simulink model "Copy_of_simpleDemonstrationDouble"  (R2023a)
settings: Solver=VariableStepAuto  StartTime=0.0  StopTime=Tstep*ofdmSymLen*6  RelTol=1e-3
PreLoadFcn:
  | % 100 MHz scenario
  | scs = 30e3;
  | fftLength = 4096;
  | NSubcarriers = 3276;
  | cpLength = 288;
  | windowLength = 20;
  | 
  | nGuardBandCarrier = fftLength - NSubcarriers;
  | ofdmSymLen = fftLength+cpLength;
  | overSamplingRate = 7;
  | filterLength = 6*70;
  | 
  | BW = scs*fftLength;                       %  Signal BW
  | Tstep = 1/BW;                   %  Simulation BW BB
  | RF = 3.7e9;                       %  RF center frequency
  | IF = 500e6;                          % IF frequency
  | dataRatePA = 1/BW;  % PA characterization sample time
  | N = nGuardBandCarrier/2;
  | HPF_cutoff = RF - 500e6;
  | 
  | bw = 100e6;
  | [txWaveform, sampleRate] = helperPACharGenerateOFDM(bw);
  | 
  | dataFileName = sprintf("helperPACharSavedData%dMHz",bw/1e6);
  | load(dataFileName,"results")
  | paInput = results.InputWaveform;
  | paOutput = results.OutputWaveform;
  | modType = 'memPoly';
  | memLen = 5;
  | degLen = 5;
  | halfDataPts = round(length(paInput)/2);
  | origState = warning;
  | warning('off', 'MATLAB:rankDeficientMatrix')
  | paModelMemPoly = double(helperPACharMemPolyModel('coefficientFinder', ...
  |   paInput(1:halfDataPts),paOutput(1:halfDataPts),memLen,degLen,modType));
  | warning(origState);
  | 
  | gain = results.LinearGain;
  | scaleFactor = double(max(abs(paOutput))/max(abs(txWaveform))/gain);
InitFcn:
  | % Initialize model parameters
  | NRInfo = get_param([gcs '/5G NR Test Model'], 'UserData');
  | MultirateBlock = [gcs '/Multirate Parameters'];
  | hInitializeNRTMModel(MultirateBlock,NRInfo);
StopFcn:
  | clear hDecodeSubframe;
undefined symbols (not defined in the file or in its folder): errorPDec, errorPInt, errorStDec, errorStInt, firceqrip, modNFloor, nDec, nInt, OSR, Probability, S, waveform
libraries: simrfV2elements x20, simrfV2util1 x11, simrfV2_lib x5, dspstat3 x4, simrfV2systems x3, commofdm x2, commrfcorlib x2, dspmlti4 x2, simrfV2junction1 x2, commrandsrc3 x1, commdigbbndam3 x1, commutil2 x1
(part 1 of 2)
settings Model: SimulationMode=accelerator  Creator=Hossein  LastModifiedBy=Hossein

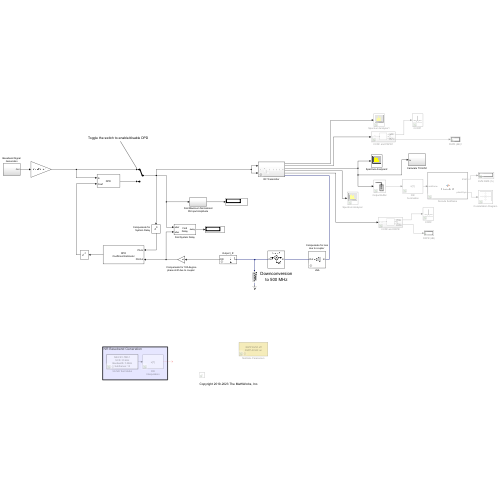
[thumbnail: Simulink's stored preview of the top-level diagram]
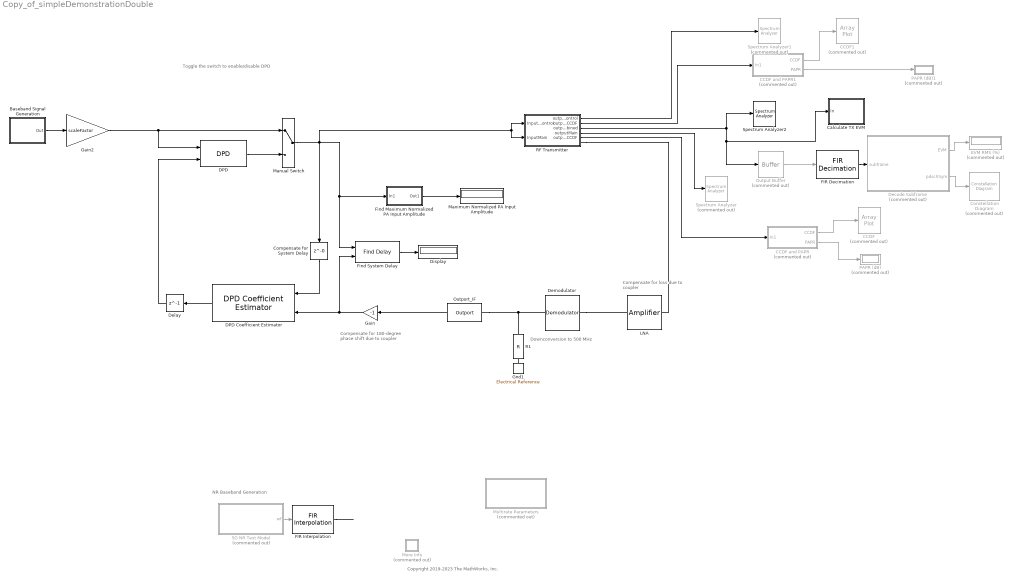
== system Copy_of_simpleDemonstrationDouble ==
  note: Copyright 2019-2023 The MathWorks, Inc.
  note: Downconversion
      | to 500 MHz
  note: Toggle the switch to enable/disable DPD
  note: Compensate for 180-degree
      | phase shift due to coupler
  note: Compensate for loss
      | due to coupler
  note: NR Baseband Generation
  5G NR Test Model : MATLAB Function  Tag=BlockGeneratedWWGApp  Commented=on  TreatAsAtomicUnit=on  SystemSampleTime=1.3020833333333333957e-07  mask(5G NR Test Model Waveform Generator){nsamps=1, OutputAfterFinalValue=Cyclic repetition}
      mask prompts: nsamps "Samples per frame:"; OutputAfterFinalValue "Form output after final data value by:"
      mask init:
      | %% Generating NR Test Models waveform
      | % NR Test Models configuration
      | cfgDLTM = nrDLCarrierConfig;
      | cfgDLTM.Label = 'NR-FR1-TM3.1';
      | cfgDLTM.FrequencyRange = 'FR1';
      | cfgDLTM.ChannelBandwidth = 5;
      | cfgDLTM.NCellID = 1;
      | cfgDLTM.NumSubframes = 10;
      | cfgDLTM.WindowingPercent = 0;
      | cfgDLTM.SampleRate = [];
      | cfgDLTM.CarrierFrequency = 0;
      | 
      | %% SCS specific carriers
      | scscarrier = nrSCSCarrierConfig;
      | scscarrier.SubcarrierSpacing = 30;
      | scscarrier.NSizeGrid = 11;
      | scscarrier.NStartGrid = 0;
      | 
      | cfgDLTM.SCSCarriers = {scscarrier};
      | 
      | %% Bandwidth Parts
      | bwp = nrWavegenBWPConfig;
      | bwp.BandwidthPartID = 1;
      | bwp.Label = 'BWP1';
      | bwp.SubcarrierSpacing = 30;
      | bwp.CyclicPrefix = 'normal';
      | bwp.NSizeBWP = 11;
      | bwp.NStartBWP = 0;
      | 
      | cfgDLTM.BandwidthParts = {bwp};
      | 
      | %% Synchronization Signals Burst
      | ssburst = nrWavegenSSBurstConfig;
      | ssburst.Enable = false;
      | ssburst.Power = 0;
      | ssburst.BlockPattern = 'Case A';
      | ssburst.TransmittedBlocks = [1 0 0 0];
      | ssburst.Period = 10;
      | ssburst.NCRBSSB = [];
      | ssburst.KSSB = 0;
      | ssburst.DataSource = 'MIB';
      | ssburst.DMRSTypeAPosition = 2;
      | ssburst.CellBarred = false;
      | ssburst.IntraFreqReselection = false;
      | ssburst.PDCCHConfigSIB1 = 0;
      | ssburst.SubcarrierSpacingCommon = 30;
      | 
      | cfgDLTM.SSBurst = ssburst;
      | 
      | %% CORESET and Search Space Configuration
      | coreset = nrCORESETConfig;
      | coreset.CORESETID = 1;
      | coreset.Label = 'CORESET1';
      | coreset.FrequencyResources = 1;
      | coreset.Duration = 2;
      | coreset.CCEREGMapping = 'noninterleaved';
      | coreset.REGBundleSize = 2;
      | coreset.InterleaverSize = 2;
      | coreset.ShiftIndex = 0;
      | coreset.PrecoderGranularity = 'sameAsREG-bundle';
      | coreset.RBOffset = [];
      | 
      | cfgDLTM.CORESET = {coreset};
      | 
      | % Search Spaces
      | searchspace = nrSearchSpaceConfig;
      | searchspace.SearchSpaceID = 1;
      | searchspace.Label = 'SearchSpace1';
      | searchspace.CORESETID = 1;
      | searchspace.SearchSpaceType = 'common';
      | searchspace.StartSymbolWithinSlot = 0;
      | searchspace.SlotPeriodAndOffset = [1 0];
      | searchspace.Duration = 1;
      | searchspace.NumCandidates = [8 8 0 0 0];
      | 
      | cfgDLTM.SearchSpaces = {searchspace};
      | 
      | %% PDCCH Instances Configuration
      | pdcch = nrWavegenPDCCHConfig;
      | pdcch.Enable = true;
      | pdcch.Label = 'PDCCH1';
      | pdcch.Power = 0;
      | pdcch.BandwidthPartID = 1;
      | pdcch.SearchSpaceID = 1;
      | pdcch.AggregationLevel = 1;
      | pdcch.AllocatedCandidate = 1;
      | pdcch.CCEOffset = [];
      | pdcch.SlotAllocation = 0;
      | pdcch.Period = 1;
      | pdcch.Coding = false;
      | pdcch.DataBlockSize = 20;
      | pdcch.DataSource = 'PN23';
      | pdcch.RNTI = 0;
      | pdcch.DMRSScramblingID = 1;
      | pdcch.DMRSPower = 0;
      | 
      | cfgDLTM.PDCCH = {pdcch};
      | 
      | %% PDSCH Instances Configuration
      | % PDSCH 1
      | pdsch1 = nrWavegenPDSCHConfig;
      | pdsch1.Enable = true;
      | pdsch1.Label = 'Partial band PDSCH sequence with 64QAM modulation scheme (target, RNTI = 0)';
      | pdsch1.Power = 0;
      | pdsch1.BandwidthPartID = 1;
      | pdsch1.Modulation = '64QAM';
      | pdsch1.NumLayers = 1;
      | pdsch1.MappingType = 'A';
      | pdsch1.ReservedCORESET = [];
      | pdsch1.SymbolAllocation = [0 14];
      | pdsch1.SlotAllocation = 0;
      | pdsch1.Period = 1;
      | pdsch1.PRBSet = 3:10;
      | pdsch1.VRBToPRBInterleaving = 0;
      | pdsch1.VRBBundleSize = 2;
      | pdsch1.NID = [];
      | pdsch1.RNTI = 0;
      | pdsch1.Coding = false;
      | pdsch1.TargetCodeRate = 0.4785;
      | pdsch1.TBScaling = 1;
      | pdsch1.XOverhead = 0;
      | pdsch1.RVSequence = 0;
      | pdsch1.DataSource = 'PN23';
      | pdsch1.DMRSPower = 0;
      | pdsch1.EnablePTRS = false;
      | pdsch1.PTRSPower = 0;
      | 
      | % PDSCH Reserved PRB
      | pdsch1ReservedPRB = nrPDSCHReservedConfig;
      | pdsch1ReservedPRB.PRBSet = 0:2;
      | pdsch1ReservedPRB.SymbolSet = [0 1];
      | pdsch1ReservedPRB.Period = 1;
      | 
      | pdsch1.ReservedPRB = {pdsch1ReservedPRB};
      | 
      | % PDSCH DM-RS
      | pdsch1DMRS = nrPDSCHDMRSConfig;
      | pdsch1DMRS.DMRSConfigurationType = 1;
      | pdsch1DMRS.DMRSReferencePoint = 'CRB0';
      | pdsch1DMRS.DMRSTypeAPosition = 2;
      | pdsch1DMRS.DMRSAdditionalPosition = 1;
      | pdsch1DMRS.DMRSLength = 1;
      | pdsch1DMRS.CustomSymbolSet = [];
      | pdsch1DMRS.DMRSPortSet = [];
      | pdsch1DMRS.NIDNSCID = [];
      | pdsch1DMRS.NSCID = 0;
      | pdsch1DMRS.NumCDMGroupsWithoutData = 1;
      | pdsch1DMRS.DMRSDownlinkR16 = 0;
      | 
      | pdsch1.DMRS = pdsch1DMRS;
      | 
      | % PDSCH PT-RS
      | pdsch1PTRS = nrPDSCHPTRSConfig;
      | pdsch1PTRS.TimeDensity = 4;
      | pdsch1PTRS.FrequencyDensity = 2;
      | pdsch1PTRS.REOffset = '00';
      | pdsch1PTRS.PTRSPortSet = [];
      | 
      | pdsch1.PTRS = pdsch1PTRS;
      | 
      | % PDSCH 2
      | pdsch2 = nrWavegenPDSCHConfig;
      | pdsch2.Enable = true;
      | pdsch2.Label = 'Partial band PDSCH sequence with 64QAM modulation scheme (target, RNTI = 2)';
      | pdsch2.Power = 0;
      | pdsch2.BandwidthPartID = 1;
      | pdsch2.Modulation = '64QAM';
      | pdsch2.NumLayers = 1;
      | pdsch2.MappingType = 'A';
      | pdsch2.ReservedCORESET = [];
      | pdsch2.SymbolAllocation = [2 12];
      | pdsch2.SlotAllocation = 0;
      | pdsch2.Period = 1;
      | pdsch2.PRBSet = 0:2;
      | pdsch2.VRBToPRBInterleaving = 0;
      | pdsch2.VRBBundleSize = 2;
      | pdsch2.NID = [];
      | pdsch2.RNTI = 2;
      | pdsch2.Coding = false;
      | pdsch2.TargetCodeRate = 0.4785;
      | pdsch2.TBScaling = 1;
      | pdsch2.XOverhead = 0;
      | pdsch2.RVSequence = 0;
      | pdsch2.DataSource = 'PN23';
      | pdsch2.DMRSPower = 0;
      | pdsch2.EnablePTRS = false;
      | pdsch2.PTRSPower = 0;
      | 
      | pdschreserved = nrPDSCHReservedConfig;
      | pdschreserved.PRBSet = 0:2;
      | pdschreserved.SymbolSet = [0 1];
      | pdschreserved.Period = 1;
      | 
      | pdsch2.ReservedPRB = {pdschreserved};
      | 
      | pdschdmrs = nrPDSCHDMRSConfig;
      | pdschdmrs.DMRSConfigurationType = 1;
      | pdschdmrs.DMRSReferencePoint = 'CRB0';
      | pdschdmrs.DMRSTypeAPosition = 2;
      | pdschdmrs.DMRSAdditionalPosition = 1;
      | pdschdmrs.DMRSLength = 1;
      | pdschdmrs.CustomSymbolSet = [];
      | pdschdmrs.DMRSPortSet = [];
      | pdschdmrs.NIDNSCID = [];
      | pdschdmrs.NSCID = 0;
      | pdschdmrs.NumCDMGroupsWithoutData = 1;
      | pdschdmrs.DMRSDownlinkR16 = 0;
      | 
      | pdsch2.DMRS = pdschdmrs;
      | 
      | pdschptrs = nrPDSCHPTRSConfig;
      | pdschptrs.TimeDensity = 4;
      | pdschptrs.FrequencyDensity = 2;
      | pdschptrs.REOffset = '00';
      | pdschptrs.PTRSPortSet = [];
      | 
      | pdsch2.PTRS = pdschptrs;
      | 
      | cfgDLTM.PDSCH = {pdsch1,pdsch2};
      | 
      | %% CSI-RS Instances Configuration
      | csirs = nrWavegenCSIRSConfig;
      | csirs.Enable = false;
      | csirs.Label = 'CSIRS1';
      | csirs.Power = 0;
      | csirs.BandwidthPartID = 1;
      | csirs.CSIRSType = 'nzp';
      | csirs.CSIRSPeriod = 'on';
      | csirs.RowNumber = 1;
      | csirs.Density = 'three';
      | csirs.SymbolLocations = 0;
      | csirs.SubcarrierLocations = 0;
      | csirs.NumRB = 11;
      | csirs.RBOffset = 0;
      | csirs.NID = 1;
      | 
      | cfgDLTM.CSIRS = {csirs};
      | 
      | % Generation
      | [waveform,info] = nrWaveformGenerator(cfgDLTM);
      | 
      | Fs = info.ResourceGrids(1).Info.SampleRate; 								 % Specify the sample rate of the waveform in Hz
      | 
      | %% Configuring block: update parameters and UserData
      | % Get current block
      | thisBlock = gcb;
      | 
      | % Set info parameters
      | maskHandle = Simulink.Mask.get(thisBlock);
      | textFsDialog = maskHandle.getDialogControl('textFs');
      | textFsDialog.Prompt = ['Waveform sample rate (Fs): ' num2str(Fs*1e-6,'%.9g') ' MHz'];
      | textWfLengthDialog = maskHandle.getDialogControl('textWFLength');
      | textWfLengthDialog.Prompt = ['Waveform length: ' num2str(length(waveform)) ' samples'];
      | 
      | % Set sample time of the block
      | set_param(thisBlock, 'SystemSampleTime', num2str(nsamps/Fs,'%.20g'));
      | 
      | % Update UserData
      | outVar.WaveformConfig = cfgDLTM;
      | outVar.WaveformLength = length(waveform);
      | outVar.Fs = Fs;
      | set_param(thisBlock, 'UserData', outVar);
  Baseband Signal Generation : Subsystem
  CCDF : ArrayPlot  Commented=on  WindowPosition=[823.000000,372.000000,866.000000,486.000000,]  ScopeFrameLocation=window  SampleIncrement=0.1  XOffset=-40.7414  YScale=Log  PlotType=Line  Title=CCDF Curve  XLabel=Rel Power (dB)  YLabel=Probability (%)  YLimits=[-12.4981,112.4829]  ShowLegend=on
  CCDF and PAPR : Subsystem  Commented=on
  CCDF and PAPR1 : Subsystem  Commented=on
  CCDF1 : ArrayPlot  Commented=on  WindowPosition=[823.000000,372.000000,866.000000,486.000000,]  ScopeFrameLocation=window  SampleIncrement=0.1  XOffset=-40.7414  YScale=Log  PlotType=Line  Title=CCDF Curve  XLabel=Rel Power (dB)  YLabel=Probability (%)  YLimits=[-12.498,112.4823]  ShowLegend=on
  Calculate TX EVM : Subsystem
  Compensate for System Delay : Delay  DelayLength=0
  Constellation Diagram : ConstellationDiagram  Commented=on  WindowPosition=[576.000000,404.000000,590.000000,412.000000,]  ScopeFrameLocation=window  ShowReferenceConstellation=off  DefaultConfigurationName=comm.scopes.ConstellationDiagramBlockCfg
  DPD : commrfcorlib/DPD  PolynomialType=Memory polynomial  CoefficientSource=Input port  Coefficients=complex([1 0 0 0 0; 0 0 0 0 0; 0 0 0 0 0])  SimulateUsing=Code generation
  DPD Coefficient Estimator : commrfcorlib/DPD Coefficient Estimator  DesiredAmplitudeGaindB=10*log10(gain)  PolynomialType=Memory polynomial  Degree=3  MemoryDepth=5  Algorithm=Recursive least squares  ForgettingFactorSource=Property  ForgettingFactor=0.999  InitialCoefficientEstimate=[]  SimulateUsing=Code generation
  Decode Subframe : MATLAB Function  Commented=on  TreatAsAtomicUnit=on
  Delay : Delay  DelayLength=1
  Demodulator : simrfV2systems/Demodulator  classname=rfdemod  Source_linear_gain=Available power gain  linear_gain=0 dB  Poly_Coeffs=[0 1]  LOFreq=RF-IF Hz  Zin=50  Zout=50  AddIRFilter=on  AddCSFilter=off  InternalGrounding=on  ForceNextInit=off  Source_Poly=Even and odd order  IPType=Input  IP2=inf dBm  IP3=inf dBm  P1dB=inf dBm  Psat=inf dBm  Gcomp=inf dBm  NF=1  Isolation=inf dB  AddPhaseNoise=off  PhaseNoiseOffset=[5e5 1e6 5e6]  PhaseNoiseLevel=[-108 -130 -140]  AutoImpulseLengthPN=on  ImpulseLengthPN=1e-10  ImpulseLength_unitPN=s  DesignMethodIR=Ideal  ResponseTypeIR=Highpass  ImplementationIR=LC Tee  ImplementationIdealIR=Constant per carrier  ImplementationRationalIR=Transfer function  UseFilterOrderIR=on  FilterOrderIR=3  PassFreq_lpIR=1  PassFreq_lp_unitIR=GHz  PassFreq_hpIR=HPF_cutoff  PassFreq_hp_unitIR=Hz  PassFreq_bpIR=[2 3]  PassFreq_bp_unitIR=GHz  PassFreq_bsIR=[1 4]  PassFreq_bs_unitIR=GHz  PassAttenIR=10*log10(2)  StopFreq_lpIR=2  StopFreq_lp_unitIR=GHz  StopFreq_hpIR=1  StopFreq_hp_unitIR=GHz  StopFreq_bpIR=[1.5 3.5]  StopFreq_bp_unitIR=GHz  StopFreq_bsIR=[2.1 2.9]  StopFreq_bs_unitIR=GHz  StopAttenIR=40  RsrcIR=50  RloadIR=50  AutoImpulseLengthIR=on  ImpulseLengthIR=1e-10  ImpulseLength_unitIR=s  DesignMethodCS=Ideal  ResponseTypeCS=Lowpass  ImplementationCS=LC Tee  ImplementationIdealCS=Constant per carrier  ImplementationRationalCS=Transfer function  UseFilterOrderCS=on  FilterOrderCS=3  PassFreq_lpCS=1  PassFreq_lp_unitCS=GHz  PassFreq_hpCS=2  PassFreq_hp_unitCS=GHz  PassFreq_bpCS=[2 3]  PassFreq_bp_unitCS=GHz  PassFreq_bsCS=[1 4]  PassFreq_bs_unitCS=GHz  PassAttenCS=10*log10(2)  StopFreq_lpCS=2  StopFreq_lp_unitCS=GHz  StopFreq_hpCS=1  StopFreq_hp_unitCS=GHz  StopFreq_bpCS=[1.5 3.5]  StopFreq_bp_unitCS=GHz  StopFreq_bsCS=[2.1 2.9]  StopFreq_bs_unitCS=GHz  StopAttenCS=40  RsrcCS=50  RloadCS=50  AutoImpulseLengthCS=on  ImpulseLengthCS=1e-10  ImpulseLength_unitCS=s
  Display : Display
  EVM RMS (%) : Display  Commented=on
  FIR Decimation : dspmlti4/FIR Decimation  FilterSource=Dialog parameters  h=firceqrip(nDec,(NRInfo.Fs*1e-6/4)/(NRInfo.Fs*1e-6*OSR/2),[errorPDec errorStDec],'passedge')  D=OSR  filtStruct=Direct form  FilterObject=FDECIM  InputProcessing=Columns as channels (frame based)  framing=Enforce single-rate processing  AllowArbitraryInputLength=off  inputOffset=0  outputBufInitCond=0  roundingMode=Floor  overflowMode=off  firstCoeffDataTypeStr=Inherit: Same word length as input  firstCoeffMin=[]  firstCoeffMax=[]  firstCoeffLastDataTypeStr=Inherit: Same word length as input  outputDataTypeStr=Inherit: Same as accumulator  outputMin=[]  outputMax=[]  outputLastDataTypeStr=Inherit: Same as accumulator
  FIR Interpolation : dspmlti4/FIR Interpolation  FilterSource=Dialog parameters  PrivateCoeffs=0  h=OSR*firceqrip(nInt,(NRInfo.Fs*1e-6/4)/(NRInfo.Fs*1e-6*OSR/2),[errorPInt errorStInt],'passedge')  L=OSR  FilterObject=FINTERP  InputProcessing=Columns as channels (frame based)  framing=Enforce single-rate processing  outputBufInitCond=0  roundingMode=Floor  overflowMode=off  firstCoeffDataTypeStr=Inherit: Same word length as input  firstCoeffMin=[]  firstCoeffMax=[]  firstCoeffLastDataTypeStr=Inherit: Same word length as input  outputDataTypeStr=Inherit: Same as accumulator  outputMin=[]  outputMax=[]  outputLastDataTypeStr=Inherit: Same as accumulator
  Find Maximum Normalized PA Input Amplitude : Subsystem
  Find System Delay : commutil2/Find Delay  corrLength=200  chgSigOP=off  stopUpdate=off  numConstDelay=3
  Gain : Gain  Gain=-1
  Gain2 : Gain  Gain=scaleFactor
  Gnd1 : simrfV2_lib/Elements/Electrical Reference
      settings: InternalSimscapePortConfiguration="{\"Bottom\":[],\"Left\":[{\"id\":\"V\",\"label\":\"\",\"type\":\"foundation.rf.circuitenvelope\"}],\"Right\":[],\"Top\":[]}"
  LNA : simrfV2elements/Amplifier  classname=amplifier  DataSource=Data file  File=unitygain.s2p  isNetworkObj=off  Paramtype=S-parameters  Sparam=[0 0;1 0]  SparamFreq=1e9 Hz  SparamZ0=50  isRationalObj=off  Residues=0  Poles=0  DF={0 0; 1 0}  Source_linear_gain=Available power gain  linear_gain=55 dB  AmAmAmPmTable=[-25,5,-1;-10,20,-2;0,27,5;5,28,12]  Zin=50  Zout=50  Source_Poly=Odd order  Poly_Coeffs=[0 1]  IPType=Output  IP2=19.5 dBm  IP3=inf dBm  P1dB=inf dBm  Psat=inf dBm  Gcomp=inf dBm  InternalGrounding=on  SourceFreq=Extracted from data source  PlotFreq=0 Hz  PlotType=X-Y plane  YParam1=S(1,1)  YFormat1=Magnitude (dB)  YParam2=None  YFormat2=Magnitude (dB)  YOption=Linear  XOption=Linear  SparamRepresentation=Time domain (rationalfit)  FitTol=-40  FitOpt=Share all poles  MaxPoles=48  AutoImpulseLength=off  ImpulseLength=0 s  MagModeling=off  AddNoise=on  NoiseType=Noise figure  NoiseDist=White  NF=0.1  MinNF=0  Gopt=0  RN=0  CarrierFreq=0 Hz  NoiseAutoImpulseLength=on  NoiseImpulseLength=1e-10 s  ConstS21NL=on  OpFreq=0 Hz  SetOpFreqAsMaxS21=on
  Manual Switch : ManualSwitch
  Maximum Normalized PA Input Amplitude : Display
  More Info : Subsystem  Commented=on
      settings: OpenFcn=showExample('5g/NRModelingAndTestingRFTransmitterExample');
      mask Display: disp('?')
  Multirate Parameters : Subsystem  Commented=on  mask{EVM3GPP=off, ACLR=on, OSR=1, nInt=45, ErrorPInt=5e-3, ErrorStInt=1e-4, nDec=45, ErrorPDec=5e-3, ErrorStDec=1e-4}
      mask prompts: EVM3GPP "Perform 3GPP EVM measurement"; ACLR "Perform 3GPP ACLR measurement"; OSR "Oversampling factor:"; nInt "Filter order:"; ErrorPInt "Maximum passband error:"; ErrorStInt "Maximum stopband error:"; nDec "Filter order:"; ErrorPDec "Maximum passband error:"; ErrorStDec "Minimum passband error:"
      mask Callback ACLR:
      | % Get handle for parameter control
      | maskHandle = Simulink.Mask.get(gcb);
      | OSRtext = maskHandle.getDialogControl('OSRText');
      | 
      | if strcmp(get_param(gcb,'ACLR'),'on')
      |      % OSR is auto
      |      maskHandle.Parameters(3).Visible = 'off';
      |      OSRtext.Visible = 'on';
      | else
      |      % OSR is user-specified
      |      maskHandle.Parameters(3).Visible = 'on';
      |      OSRtext.Visible = 'off';
      | end
      mask DialogControl Container4 Prompt: Multirate Parameters
      mask DialogControl Control1 Prompt: Parameters to configure the example measurements and the FIR Interpolation and Decimation blocks. These blocks resample and filter the waveform to allow you to see the effect of the high power amplifier on the out of band spectral emissions. If the 3GPP ACLR measurement is enabled, then the oversampling factor is calculated during run time according to the 3GPP specifications. If the 3GPP EVM measurement is enabled, EVM measurement for PDSCH is done using the 3GPP specified EVM algorithm as defined in TS 38.104, Annex B(FR1) / Annex C(FR2).
      mask DialogControl DescGroupVar Prompt: Measurement Parameters
      mask DialogControl OSRText Prompt: Oversampling factor calculated during run time.
      mask DialogControl Container2 Prompt: FIR Interpolation Parameters
      mask DialogControl Container3 Prompt: FIR Decimation Parameters
      mask Display:
      | % Display the parameters on the mask icon
      | block = [gcs '/Multirate Parameters'];
      | ACLR = get_param(block,'ACLR');
      | EVM = get_param(block,'EVM3GPP');
      | str = ['3GPP EVM: ' EVM '\n'...
      |        '3GPP ACLR: ' ACLR];
      | fprintf(str);
  Outport_IF : simrfV2util1/Outport  SensorType=Ideal voltage  OutputFormat=Complex Baseband  CarrierFreq=IF Hz  ZL=Inf  InternalGrounding=on  StepSize=-1 s  AutoStep=off  HalfPolyphaseLength=0
  Output Buffer : Buffer  Commented=on  N=NRInfo.WaveformLength/NRInfo.WaveformConfig.NumSubframes*OSR  OutputFrames=off
  PAPR (dB) : Display  Commented=on
  PAPR (dB)1 : Display  Commented=on
  R1 : simrfV2elements/R  classname=resistor  Resistance=50 Ohm  AddNoise=on
  RF Transmitter : Subsystem  mask(RF Transmitter){carrierFreq=2140, ifFreq=70, sourceImpedance=50, loadImpedance=50, temperature=290, modGain=-6, loFreq=[], modGainMismatch=0, modPhaseMismatch=0, modIsolation=26.7, modImpedance=50, modIP3=26, modNFloor=modNFloor, modPNOffset=[3.75e3 10e3 100e3 1e6], modPNLevel=[-80.1 -95.7 -118.6 -139.2], impulseDuration=2.5e-4, bpFilterPassFreq=[2050 2230], bpFilterPassAtten=1.1, bpFilterStopFreq=[1550 2730], bpFilterStopAtten=31, bpFilterImpedance=50, vgaGain=0, vgaNF=2, vgaIP3=47, vgaP1dB=35, vgaImpedance=50, hpaGain=25, hpaNF=7, hpaIP3=47, hpaP1dB=35, hpaImpedance=50}
      mask prompts: carrierFreq "Center frequency (MHz):"; ifFreq "Intermediate frequency (MHz):"; sourceImpedance "Source impedance (Ohm):"; loadImpedance "Load impedance (Ohm):"; temperature "System temperature (K):"; modGain "Gain (dB):"; loFreq "LO frequency (MHz):"; modGainMismatch "I/Q gain mismatch (dB):"; modPhaseMismatch "I/Q phase mismatch (Deg):"; modIsolation "LO to RF isolation (dB):"; modImpedance "Impedance (Ohm):"; modIP3 "IP3 (dBm):"; modNFloor "Noise floor (dBm/Hz):"; modPNOffset "Phase noise offset (Hz):"; modPNLevel "Phase noise level (dBc/Hz):"; impulseDuration "Impulse response duration (s):"; bpFilterPassFreq "Passband frequencies (MHz):"; bpFilterPassAtten "Passband attenuation (dB):"; bpFilterStopFreq "Stopband frequencies (MHz):"; bpFilterStopAtten "Stopband attenuation (dB):"; bpFilterImpedance "Impedance (Ohm)"; vgaGain "Gain (0-20 dB):"; vgaNF "Noise figure (dB):"; vgaIP3 "IP3 (dBm):"; vgaP1dB "P1dB (dBm):"; vgaImpedance "Impedance (Ohm)"; hpaGain "Gain (dB):"; hpaNF "Noise figure (dB):"; hpaIP3 "IP3 (dBm):"; hpaP1dB "P1dB (dBm):"; hpaImpedance "Impedance (Ohm)"
      mask help: Estimate the impact of non-linearity, phase noise, impedance mismatch and IQ imbalance.
      mask init:
      | modNFloor = 10*log10(1.381e-23*temperature*1000);
      | loFreq = carrierFreq-ifFreq;
      mask Help:
      | This architecture upconverts the waveform to the carrier frequency 2140MHz (default) and applies RF filtering and amplification before transmitting the signal. RF impairments such as non-linearity, phase noise, impedance mismatch and IQ imbalance are introduced by the RF chain, which is composed by an IQ modulator, a bandpass filter, a VGA and an HPA.
      | 
      | This subsystem uses components from the RF Blockset Circuit Envelope library.
      mask DialogControl Container12 Prompt: RF Stage
      mask DialogControl Container20 Prompt: Radio Frequency Stage Parameters
      mask DialogControl Container7 Prompt: IQ Modulator
      mask DialogControl Container8 Prompt: Up-Conversion Characteristics
      mask DialogControl Container13 Prompt: BP Filter
      mask DialogControl Container11 Prompt: Bandpass Filter Characteristics
      mask DialogControl Container16 Prompt: VGA
      mask DialogControl Container19 Prompt: Variable Gain Amplifier Characteristics at Center Frequency
      mask DialogControl Container14 Prompt: HPA
      mask DialogControl Container15 Prompt: High Power Amplifier Characteristics at Center Frequency
      mask Display:
      | % Use specified image as mask icon
      | image('RFTransmitterRFIcon.png')
  Spectrum Analyzer : SpectrumAnalyzer  Commented=on  WindowPosition=[487.000000,397.000000,1016.000000,517.000000,]  ScopeFrameLocation=window  SampleRate=30720000  Span=30720000.000000004  StartFrequency=-15360000.000000002  StopFrequency=15360000.000000002  RBWSource=Property  RBW=30000  ForgettingFactor=0.99388  VBWSource=Property  VBW=3000  YLimits=[-102.46917614,8.54977013]
  Spectrum Analyzer1 : SpectrumAnalyzer  Commented=on  WindowPosition=[487.000000,397.000000,1016.000000,517.000000,]  ScopeFrameLocation=window  SampleRate=30720000  Span=30720000.000000004  StartFrequency=-15360000.000000002  StopFrequency=15360000.000000002  RBWSource=Property  RBW=30000  ForgettingFactor=0.99388  VBWSource=Property  VBW=3000  YLimits=[-102.46917614,8.54977013]
  Spectrum Analyzer2 : SpectrumAnalyzer  WindowPosition=[792.000000,194.000000,1016.000000,517.000000,]  Visible=on  ScopeFrameLocation=window  SampleRate=30720000  Span=30720000.000000004  StartFrequency=-15360000.000000002  StopFrequency=15360000.000000002  RBWSource=Property  RBW=30000  ForgettingFactor=0.99388  VBWSource=Property  VBW=3000  YLimits=[-102.46917614,8.54977013]
  wires:
  CCDF and PAPR/2(PAPR) -> PAPR (dB)/1
  Manual Switch/1 -> RF Transmitter/1(InputControl), RF Transmitter/2(InputMain), Compensate for System Delay/1, Find System Delay/1, Find Maximum Normalized PA Input Amplitude/1(In1)
  CCDF and PAPR/1(CCDF) -> CCDF/1
  Output Buffer/1 -> FIR Decimation/1
  Decode Subframe/2(pdschSym) -> Constellation Diagram/1
  Decode Subframe/1(EVM) -> EVM RMS (%)/1
  FIR Decimation/1 -> Decode Subframe/1(subframe)
  RF Transmitter/5(outputMainCCDF) -> CCDF and PAPR/1(In1)
  Gain/1 -> Find System Delay/2, DPD Coefficient Estimator/2
  DPD Coefficient Estimator/1 -> Delay/1
  Gain2/1 -> DPD/1, Manual Switch/1
  DPD/1 -> Manual Switch/2
  Compensate for System Delay/1 -> DPD Coefficient Estimator/1
  Find Maximum Normalized PA Input Amplitude/1(Out1) -> Maximum Normalized PA Input Amplitude/1
  Delay/1 -> DPD/2
  Outport_IF/1 -> Gain/1
  Find System Delay/1 -> Display/1
  CCDF and PAPR1/2(PAPR) -> PAPR (dB)1/1
  CCDF and PAPR1/1(CCDF) -> CCDF1/1
  RF Transmitter/2(outputControlCCDF) -> CCDF and PAPR1/1(In1)
  RF Transmitter/4(outputMain) -> Spectrum Analyzer/1
  RF Transmitter/1(outputControl) -> Spectrum Analyzer1/1
  FIR Interpolation/1 -> ?
  5G NR Test Model/1(wf) -> FIR Interpolation/1
  Baseband Signal Generation/1(Out) -> Gain2/1
  RF Transmitter/3(outputCombined) -> Calculate TX EVM/1(In), Output Buffer/1, Spectrum Analyzer2/1
  connections:
  R1/LConn1 -- Outport_IF/LConn1 -- Demodulator/RConn1
  Demodulator/LConn1 -- LNA/RConn1
  RF Transmitter/RConn1 -- LNA/LConn1
  Gnd1/LConn1 -- R1/RConn1

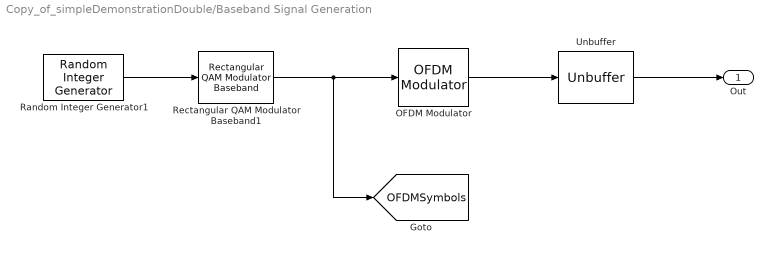
== system Copy_of_simpleDemonstrationDouble/Baseband Signal Generation ==
  OFDM Modulator : commofdm/OFDM Modulator  FFTLength=fftLength  NumGuardBandCarriers=[N+1; N]  InsertDCNull=off  PilotInputPort=off  PilotCarrierIndices=[12; 26; 40; 54]  CyclicPrefixLength=cpLength  Windowing=on  WindowLength=windowLength  OversamplingFactor=overSamplingRate  NumSymbols=1  NumTransmitAntennas=1  SimulateUsing=Code generation
  Random Integer Generator1 : commrandsrc3/Random Integer Generator  SetSize=64  SeedSource=Parameter  Seed=242  SampleTime=Tstep*(ofdmSymLen/(fftLength-2*N-1))  SamplesPerFrame=fftLength-2*N-1  OutputDataType=double  SimulateUsing=Code generation
  Rectangular QAM Modulator Baseband1 : commdigbbndam3/Rectangular QAM Modulator Baseband  M=64  InType=Integer  Enc=Gray  Mapping=[0:15]  PowType=Min. distance between symbols  MinDist=2  AvgPow=1  PeakPow=1  Ph=0  outDtype=double  outWordLen=16  outUDDataType=sfix(16)  outFracLenMode=Best precision  outFracLen=15  outDataTypeStr=double  outLastDataTypeStr=double
  Unbuffer : Unbuffer
  Out : Outport  VectorParamsAs1DForOutWhenUnconnected=off
  tag scope: OFDMSymbols=global
  wires:
  Random Integer Generator1/1 -> Rectangular QAM Modulator Baseband1/1
  Unbuffer/1 -> Out/1
  Rectangular QAM Modulator Baseband1/1 -> [OFDMSymbols], OFDM Modulator/1
  OFDM Modulator/1 -> Unbuffer/1

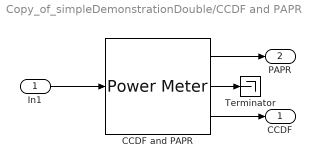
== system Copy_of_simpleDemonstrationDouble/CCDF and PAPR ==
  In1 : Inport
  CCDF and PAPR : dspstat3/Power Meter  Measurement=Peak-to-average power ratio  ReferenceLoad=1  OutputPowerUnits=dBm  WindowLength=256  OverlapLength=255  AllowArbitraryInputLength=off  ComputeCCDF=on  PowerRange=50  PowerResolution=0.1  CCDFOutput=Relative power and probability (whole CCDF curve)  ProbabilityVector=[ 10; 1; 0.1; 0.01; 0.001; 0.0001 ]  RelativePowerVector=[ 0; 3; 6; 9; 12 ]  ResetPort=off  SimulateUsing=Code generation
  Terminator : Terminator
  CCDF : Outport
  PAPR : Outport  Port=2
  wires:
  In1/1 -> CCDF and PAPR/1
  CCDF and PAPR/3 -> CCDF/1
  CCDF and PAPR/2 -> Terminator/1
  CCDF and PAPR/1 -> PAPR/1

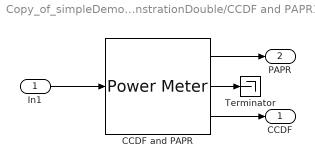
== system Copy_of_simpleDemonstrationDouble/CCDF and PAPR1 ==
  In1 : Inport
  CCDF and PAPR : dspstat3/Power Meter  Measurement=Peak-to-average power ratio  ReferenceLoad=1  OutputPowerUnits=dBm  WindowLength=256  OverlapLength=255  AllowArbitraryInputLength=off  ComputeCCDF=on  PowerRange=50  PowerResolution=0.1  CCDFOutput=Relative power and probability (whole CCDF curve)  ProbabilityVector=[ 10; 1; 0.1; 0.01; 0.001; 0.0001 ]  RelativePowerVector=[ 0; 3; 6; 9; 12 ]  ResetPort=off  SimulateUsing=Code generation
  Terminator : Terminator
  CCDF : Outport
  PAPR : Outport  Port=2
  wires:
  In1/1 -> CCDF and PAPR/1
  CCDF and PAPR/3 -> CCDF/1
  CCDF and PAPR/2 -> Terminator/1
  CCDF and PAPR/1 -> PAPR/1

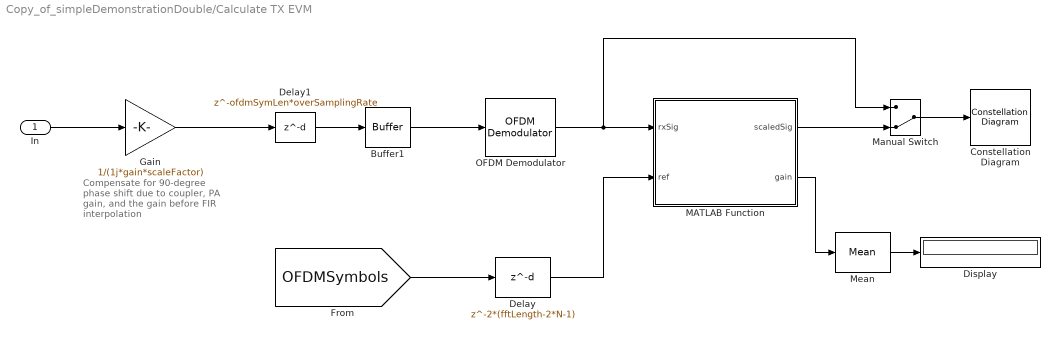
== system Copy_of_simpleDemonstrationDouble/Calculate TX EVM ==
  note: Compensate for 90-degree
      | phase shift due to coupler,
      | PA gain, and the gain before
      | FIR interpolation
  In : Inport
  Buffer1 : Buffer  N=ofdmSymLen*overSamplingRate  OutputFrames=off
  Constellation Diagram : ConstellationDiagram  WindowPosition=[501.000000,93.000000,973.000000,546.000000,]  Visible=on  ScopeFrameLocation=window  ReferenceConstellation="{[-7+7i  -7+5i  -7+3i  -7+1i  -7-1i  -7-3i  -7-5i  -7-7i  -5+7i  -5+5i  -5+3i  -5+1i  -5-1i  -5-3i  -5-5i  -5-7i  -3+7i  -3+5i  -3+3i  -3+1i  -3-1i  -3-3i  -3-5i  -3-7i  -1+7i  -1+5i  -1+3i  -1+1i  -1-1i  -1-3i  -1-5i  -1-7i   1+7i   1+5i   1+3i   1+1i   1-1i   1-3i   1-5i   1-7i   3+7i   3+5i   3+3i   3+1i   3-1i   3-3i   3-5i   3-7i   5+7i   5+5i   5+3i   5+1i   5-1i   5-3i   5-5i   5-7i   7+7i   7+5i   7+3i   7+1i   7-1i   7-3i   7-5i   7-7i]}"  XLimits=[-9.7559 9.963]  YLimits=[-9.7559 9.963]  EnableMeasurements=on  DefaultConfigurationName=comm.scopes.ConstellationDiagramBlockCfg
  Delay : Delay  DelayLength=2*(fftLength-2*N-1)  InputProcessing=Columns as channels (frame based)
  Delay1 : Delay  DelayLength=ofdmSymLen*overSamplingRate  InputProcessing=Columns as channels (frame based)
  Display : Display
  Gain : Gain  Gain=1/(1j*gain*scaleFactor)
  MATLAB Function : MATLAB Function  TreatAsAtomicUnit=on
  Manual Switch : ManualSwitch  CurrentSetting=0
  Mean : dspstat3/Mean  run=off  InputProcessing=Columns as channels (frame based)  reset_popup=None  directionMode=Each column  dimension=1  roiEnable=off  roiType=Rectangles  roiPortion=Entire ROI  roiOutput=Individual statistics for each ROI  roiFlag=off  roundingMode=Floor  overflowMode=off  outputDataTypeStr=Inherit: Same as accumulator  outputMin=[]  outputMax=[]  outputLastDataTypeStr=Inherit: Same as accumulator
  OFDM Demodulator : commofdm/OFDM Demodulator  FFTLength=fftLength  NumGuardBandCarriers=[N+1; N]  RemoveDCCarrier=off  PilotOutputPort=off  PilotCarrierIndices=[12; 26; 40; 54]  CyclicPrefixLength=cpLength  OversamplingFactor=overSamplingRate  NumSymbols=1  NumReceiveAntennas=1  SimulateUsing=Code generation
  wires:
  Buffer1/1 -> OFDM Demodulator/1
  In/1 -> Gain/1
  MATLAB Function/2(gain) -> Mean/1
  MATLAB Function/1(scaledSig) -> Manual Switch/2
  Manual Switch/1 -> Constellation Diagram/1
  OFDM Demodulator/1 -> MATLAB Function/1(rxSig), Manual Switch/1
  [OFDMSymbols] -> Delay/1
  Delay/1 -> MATLAB Function/2(ref)
  Mean/1 -> Display/1
  Gain/1 -> Delay1/1
  Delay1/1 -> Buffer1/1

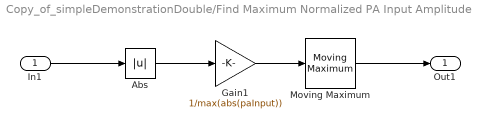
== system Copy_of_simpleDemonstrationDouble/Find Maximum Normalized PA Input Amplitude ==
  In1 : Inport
  Abs : Abs  SaturateOnIntegerOverflow=off
  Gain1 : Gain  Gain=1/max(abs(paInput))
  Moving Maximum : dspstat3/Moving Maximum  SpecifyWindowLength=off  WindowLength=4  SimulateUsing=Code generation
  Out1 : Outport
  wires:
  Abs/1 -> Gain1/1
  Gain1/1 -> Moving Maximum/1
  Moving Maximum/1 -> Out1/1
  In1/1 -> Abs/1

== system Copy_of_simpleDemonstrationDouble/More Info ==

== system Copy_of_simpleDemonstrationDouble/Multirate Parameters ==
